simulink model "hardware_motor_arduino"  (R2020b)
settings: Solver=FixedStepAuto  StartTime=0.0  StopTime=inf  FixedStep=0.04  RelTol=1e-3  EnableMultiTasking=on
libraries: arduinolib x8
settings Model: SILPILModeSetting=veronly  ExtModeTrigDuration=2  Creator=ASUS  LastModifiedBy=ONLY-GOD
settings OptimizationCC: EnhancedBackFolding=on  PassReuseOutputArgsAs=Individual arguments  ZeroExternalMemoryAtStartup=off  ZeroInternalMemoryAtStartup=off  MaxStackSize=64  OptimizeBlockOrder=speed  DifferentSizesBufferReuse=on  OptimizationCustomize=off  EfficientTunableParamExpr=on
settings DebuggingCC: ParameterTunabilityLossMsg=error
settings HardwareCC: ProdBitPerPointer=32  ProdBitPerSizeT=32  ProdBitPerPtrDiffT=32  ProdLargestAtomicInteger=Long  ProdLargestAtomicFloat=Double  ProdWordSize=32  ProdHWDeviceType=ARM Compatible->ARM Cortex
settings SFSimCC: MATLABDynamicMemAlloc=off
settings RTWCC: Description=Embedded Coder  SystemTargetFile=ert.tlc  HardwareBoard=Arduino Due  TemplateMakefile=ert_default_tmf  Toolchain=Arduino ARM  BuildConfiguration=Faster Runs
settings CodeAppCC: ForceParamTrailComments=on  IgnoreCustomStorageClasses=off  OperatorAnnotations=on  SimulinkDataObjDesc=on  SFDataObjDesc=on  InsertBlockDesc=on
settings ERTTargetCC: SupportContinuousTime=on  SupportVariableSizeSignals=on  ExtModeTransport=3  ExtModeStaticAllocSize=24576  ExtModeMexFile=ext_xcp  ExtModeIntrfLevel=Level2 - Open

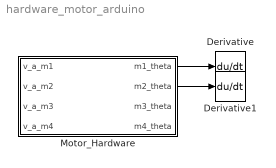
== system hardware_motor_arduino ==
  Derivative : Derivative
  Derivative1 : Derivative
  Motor_Hardware : Subsystem
  wires:
  Motor_Hardware/1(m1_theta) -> Derivative/1
  Motor_Hardware/2(m2_theta) -> Derivative1/1

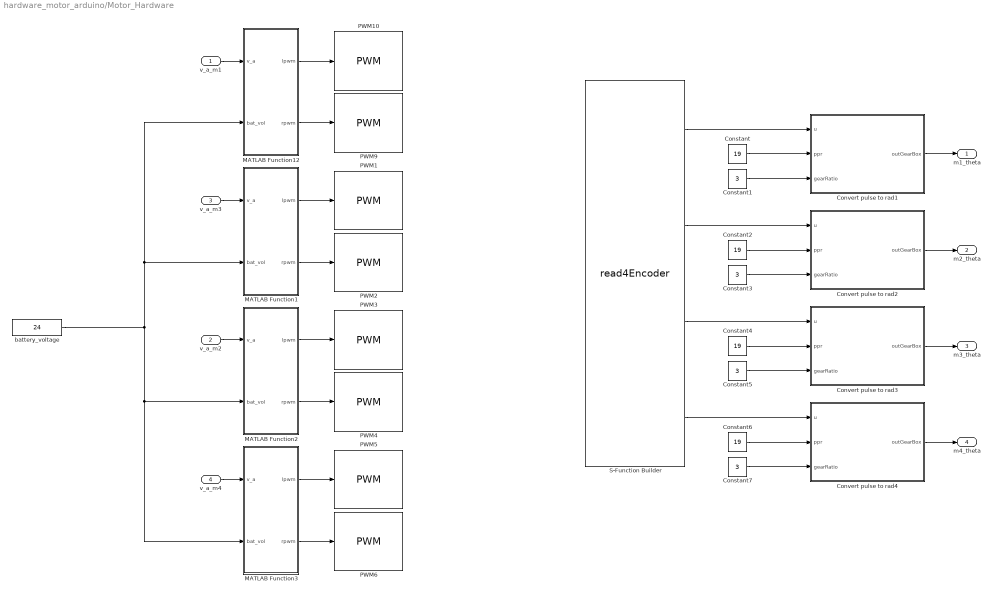
== system hardware_motor_arduino/Motor_Hardware ==
  v_a_m1 : Inport
  v_a_m2 : Inport  Port=2
  v_a_m3 : Inport  Port=3
  v_a_m4 : Inport  Port=4
  Constant{,2,4,6} (4 alike) : Constant  Value=19
  Constant{1,3,5,7} (4 alike) : Constant  Value=3
  Convert pulse to rad1 : MATLAB Function  TreatAsAtomicUnit=on
  Convert pulse to rad2 : MATLAB Function  TreatAsAtomicUnit=on
  Convert pulse to rad3 : MATLAB Function  TreatAsAtomicUnit=on
  Convert pulse to rad4 : MATLAB Function  TreatAsAtomicUnit=on
  MATLAB Function1 : MATLAB Function  TreatAsAtomicUnit=on
  MATLAB Function12 : MATLAB Function  TreatAsAtomicUnit=on
  MATLAB Function2 : MATLAB Function  TreatAsAtomicUnit=on
  MATLAB Function3 : MATLAB Function  TreatAsAtomicUnit=on
  PWM1 : arduinolib/PWM  pinNumber=5  frequencyType=Default  desiredFrequency=490.2  achievableFrequency=490.2
  PWM10 : arduinolib/PWM  pinNumber=7  frequencyType=Default  desiredFrequency=490.2  achievableFrequency=490.2
  PWM2 : arduinolib/PWM  pinNumber=4  frequencyType=Default  desiredFrequency=490.2  achievableFrequency=490.2
  PWM3 : arduinolib/PWM  pinNumber=12  frequencyType=Default  desiredFrequency=490.2  achievableFrequency=490.2
  PWM4 : arduinolib/PWM  pinNumber=13  frequencyType=Default  desiredFrequency=490.2  achievableFrequency=490.2
  PWM5 : arduinolib/PWM  pinNumber=3  frequencyType=Default  desiredFrequency=490.2  achievableFrequency=490.2
  PWM6 : arduinolib/PWM  pinNumber=2  frequencyType=Default  desiredFrequency=490.2  achievableFrequency=490.2
  PWM9 : arduinolib/PWM  pinNumber=6  frequencyType=Default  desiredFrequency=490.2  achievableFrequency=490.2
  S-Function Builder : S-Function  FunctionName=read4Encoder  SFunctionModules=read4Encoder_wrapper  SFunctionDeploymentMode=off  EnableBusSupport=off  mask(S-Function Builder){}
      mask help: Simulink:masks:SFunctionBuilder_MD
      mask init:
      | val = [[.9  0.75 0.75 1 1 .9 .9 1]',[1 1 0.75 0.75 .9 .9 1 .9]'];try , sys = get_param(gcb,'SfunBuilderFcnName');if isempty(sys), sys = get_param(gcb,'FunctionName'); end,catch, sys = get_param(gcb,'FunctionName'); end
      settings: CopyFcn=set_param(gcbh,'LinkStatus','none')  OpenFcn=sfunctionwizard(gcbh)
      mask Display: plot(val(:,1),val(:,2)),disp(sys),port_label('output',1,'count1'),port_label('output',2,'count2'),port_label('output',3,'count3'),port_label('output',4,'count4')
  battery_voltage : Constant  Value=24
  m1_theta : Outport
  m2_theta : Outport  Port=2
  m3_theta : Outport  Port=3
  m4_theta : Outport  Port=4
  wires:
  MATLAB Function12/2(rpwm) -> PWM9/1
  MATLAB Function12/1(lpwm) -> PWM10/1
  v_a_m1/1 -> MATLAB Function12/1(v_a)
  Constant/1 -> Convert pulse to rad1/2(ppr)
  Constant1/1 -> Convert pulse to rad1/3(gearRatio)
  Constant3/1 -> Convert pulse to rad2/3(gearRatio)
  Constant2/1 -> Convert pulse to rad2/2(ppr)
  Constant5/1 -> Convert pulse to rad3/3(gearRatio)
  Constant4/1 -> Convert pulse to rad3/2(ppr)
  Constant7/1 -> Convert pulse to rad4/3(gearRatio)
  Constant6/1 -> Convert pulse to rad4/2(ppr)
  MATLAB Function1/1(lpwm) -> PWM1/1
  MATLAB Function1/2(rpwm) -> PWM2/1
  MATLAB Function2/1(lpwm) -> PWM3/1
  MATLAB Function2/2(rpwm) -> PWM4/1
  MATLAB Function3/1(lpwm) -> PWM5/1
  MATLAB Function3/2(rpwm) -> PWM6/1
  S-Function Builder/1 -> Convert pulse to rad1/1(u)
  S-Function Builder/2 -> Convert pulse to rad2/1(u)
  S-Function Builder/3 -> Convert pulse to rad3/1(u)
  S-Function Builder/4 -> Convert pulse to rad4/1(u)
  v_a_m3/1 -> MATLAB Function1/1(v_a)
  v_a_m2/1 -> MATLAB Function2/1(v_a)
  v_a_m4/1 -> MATLAB Function3/1(v_a)
  battery_voltage/1 -> MATLAB Function12/2(bat_vol), MATLAB Function1/2(bat_vol), MATLAB Function2/2(bat_vol), MATLAB Function3/2(bat_vol)
  Convert pulse to rad1/1(outGearBox) -> m1_theta/1
  Convert pulse to rad2/1(outGearBox) -> m2_theta/1
  Convert pulse to rad3/1(outGearBox) -> m3_theta/1
  Convert pulse to rad4/1(outGearBox) -> m4_theta/1

== matlab function hardware_motor_arduino/Motor_Hardware/Convert pulse to rad1 ==
  settings: updateMethod=DISCRETE
  data: u input; ppr input; gearRatio input; outGearBox output
function outGearBox = fcn(u,ppr,gearRatio)

persistent counter_num over_flag
if(isempty(counter_num)), counter_num = 0;end
if(isempty(over_flag)), over_flag = 0;end
pulse2radian = 2*pi/ppr; % 1 pulse = ?? radian

if(double(u) - counter_num > 40000), over_flag = over_flag-1;
elseif(double(u) - counter_num < -40000), over_flag = over_flag+1;
end

inGearBox = (double(u)+over_flag*(2^32 -1))*pulse2radian; 
outGearBox = inGearBox/gearRatio;
counter_num = double(u) ;

== matlab function hardware_motor_arduino/Motor_Hardware/Convert pulse to rad2 ==
  settings: updateMethod=DISCRETE
  data: u input; ppr input; gearRatio input; outGearBox output
function outGearBox = fcn(u,ppr,gearRatio)

persistent counter_num over_flag
if(isempty(counter_num)), counter_num = 0;end
if(isempty(over_flag)), over_flag = 0;end
pulse2radian = 2*pi/ppr; % 1 pulse = ?? radian

if(double(u) - counter_num > 40000), over_flag = over_flag-1;
elseif(double(u) - counter_num < -40000), over_flag = over_flag+1;
end

inGearBox = (double(u)+over_flag*(2^32 -1))*pulse2radian; 
outGearBox = inGearBox/gearRatio;
counter_num = double(u) ;

== matlab function hardware_motor_arduino/Motor_Hardware/Convert pulse to rad3 ==
  settings: updateMethod=DISCRETE
  data: u input; ppr input; gearRatio input; outGearBox output
function outGearBox = fcn(u,ppr,gearRatio)

persistent counter_num over_flag
if(isempty(counter_num)), counter_num = 0;end
if(isempty(over_flag)), over_flag = 0;end
pulse2radian = 2*pi/ppr; % 1 pulse = ?? radian

if(double(u) - counter_num > 40000), over_flag = over_flag-1;
elseif(double(u) - counter_num < -40000), over_flag = over_flag+1;
end

inGearBox = (double(u)+over_flag*(2^32 -1))*pulse2radian; 
outGearBox = inGearBox/gearRatio;
counter_num = double(u) ;

== matlab function hardware_motor_arduino/Motor_Hardware/Convert pulse to rad4 ==
  settings: updateMethod=DISCRETE
  data: u input; ppr input; gearRatio input; outGearBox output
function outGearBox = fcn(u,ppr,gearRatio)

persistent counter_num over_flag
if(isempty(counter_num)), counter_num = 0;end
if(isempty(over_flag)), over_flag = 0;end
pulse2radian = 2*pi/ppr; % 1 pulse = ?? radian

if(double(u) - counter_num > 40000), over_flag = over_flag-1;
elseif(double(u) - counter_num < -40000), over_flag = over_flag+1;
end

inGearBox = (double(u)+over_flag*(2^32 -1))*pulse2radian; 
outGearBox = inGearBox/gearRatio;
counter_num = double(u) ;

== matlab function hardware_motor_arduino/Motor_Hardware/MATLAB Function1 ==
  data: v_a input; lpwm output; rpwm output; bat_vol input
function [lpwm,rpwm] = fcn(v_a,bat_vol)

pwm = v_a*255/bat_vol;
if pwm > 0
    lpwm = pwm;
    rpwm = 0;
elseif pwm < 0
    lpwm = 0;
    rpwm = abs(pwm);
else
    lpwm = 0;
    rpwm = 0;
end

== matlab function hardware_motor_arduino/Motor_Hardware/MATLAB Function2 ==
  data: v_a input; lpwm output; rpwm output; bat_vol input
function [lpwm,rpwm] = fcn(v_a,bat_vol)

pwm = v_a*255/bat_vol;
if pwm > 0
    lpwm = pwm;
    rpwm = 0;
elseif pwm < 0
    lpwm = 0;
    rpwm = abs(pwm);
else
    lpwm = 0;
    rpwm = 0;
end

== matlab function hardware_motor_arduino/Motor_Hardware/MATLAB Function3 ==
  data: v_a input; lpwm output; rpwm output; bat_vol input
function [lpwm,rpwm] = fcn(v_a,bat_vol)

pwm = v_a*255/bat_vol;
if pwm > 0
    lpwm = pwm;
    rpwm = 0;
elseif pwm < 0
    lpwm = 0;
    rpwm = abs(pwm);
else
    lpwm = 0;
    rpwm = 0;
end

== matlab function hardware_motor_arduino/Motor_Hardware/MATLAB Function12 ==
  data: v_a input; lpwm output; rpwm output; bat_vol input
function [lpwm,rpwm] = fcn(v_a,bat_vol)

pwm = v_a*255/bat_vol;
if pwm > 0
    lpwm = pwm;
    rpwm = 0;
elseif pwm < 0
    lpwm = 0;
    rpwm = abs(pwm);
else
    lpwm = 0;
    rpwm = 0;
end
